simulink library "INT_OilT_VD"  (R2016b)
settings: Solver=VariableStepAuto  StartTime=0.0  StopTime=10.0  RelTol=1e-3
settings Model: Creator=Administrator  LastModifiedBy=Administrator

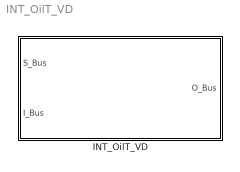
== system INT_OilT_VD ==
  INT_OilT_VD : Subsystem

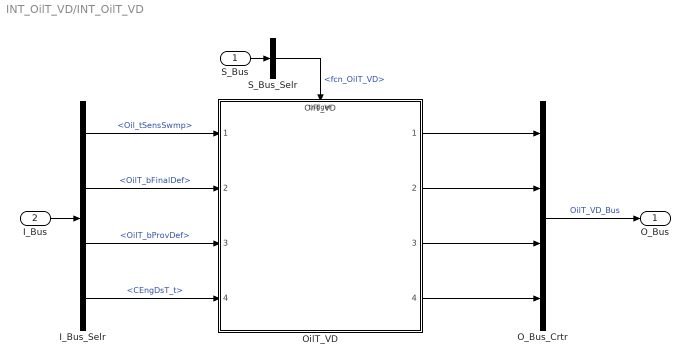
== system INT_OilT_VD/INT_OilT_VD ==
  S_Bus : Inport
  I_Bus : Inport  Port=2
  I_Bus_Selr : BusSelector  OutputSignals=Oil_tSensSwmp,OilT_bFinalDef,OilT_bProvDef,CEngDsT_t
  O_Bus_Crtr : BusCreator  Inputs=4
  OilT_VD : ModelReference  ModelNameDialog=OilT_VD  SimulationMode=Normal  ModelReferenceVersion=1.6  TriggerPortName=function  TriggerPortTriggerType=function-call  TriggerPortStatesWhenEnabling=held
  S_Bus_Selr : BusSelector  OutputSignals=fcn_OilT_VD
  O_Bus : Outport
  wires:
  S_Bus_Selr/1 -> OilT_VD/Trigger  "<fcn_OilT_VD>"
  S_Bus/1 -> S_Bus_Selr/1
  I_Bus/1 -> I_Bus_Selr/1
  I_Bus_Selr/1 -> OilT_VD/1  "<Oil_tSensSwmp>"
  I_Bus_Selr/2 -> OilT_VD/2  "<OilT_bFinalDef>"
  I_Bus_Selr/3 -> OilT_VD/3  "<OilT_bProvDef>"
  I_Bus_Selr/4 -> OilT_VD/4  "<CEngDsT_t>"
  O_Bus_Crtr/1 -> O_Bus/1  "OilT_VD_Bus"
  OilT_VD/1 -> O_Bus_Crtr/1
  OilT_VD/2 -> O_Bus_Crtr/2
  OilT_VD/3 -> O_Bus_Crtr/3
  OilT_VD/4 -> O_Bus_Crtr/4
